simulink model "sat_CH_MC_v7"  (R2017b)
settings: Solver=VariableStepAuto  StartTime=0.0  StopTime=2000  RelTol=1e-5
settings Model: Creator=J  LastModifiedBy=student

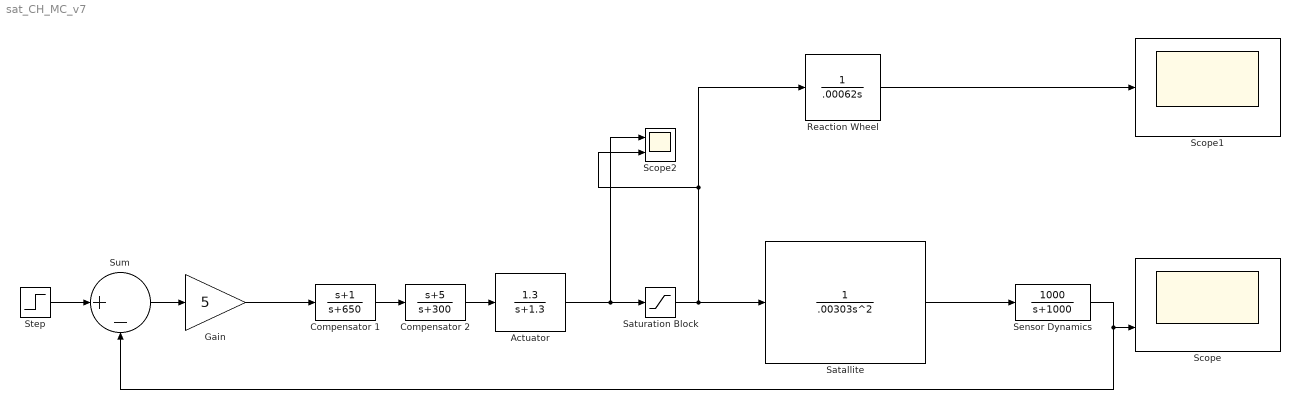
== system sat_CH_MC_v7 ==
  Actuator : TransferFcn  Numerator=[1.3]  Denominator=[1 1.3]
  Compensator 1 : TransferFcn  Numerator=[1 1]  Denominator=[1 650]
  Compensator 2 : TransferFcn  Numerator=[1 5]  Denominator=[1 300]
  Gain : Gain  Gain=5
  Reaction Wheel : TransferFcn  Denominator=[.00062 0]
  Satallite : TransferFcn  Denominator=[.00303 0 0]
  Saturation Block : Saturate  UpperLimit=.007  LowerLimit=-.007
  Scope : Scope  NumInputPorts=2
  Scope1 : Scope
  Scope2 : Scope  NumInputPorts=2
  Sensor Dynamics : TransferFcn  Numerator=[1000]  Denominator=[1 1000]
  Step : Step  SampleTime=0
  Sum : Sum  Inputs=|+-
  wires:
  Actuator/1 -> Scope2/1, Saturation Block/1
  Sum/1 -> Gain/1
  Step/1 -> Sum/1
  Saturation Block/1 -> Satallite/1, Reaction Wheel/1, Scope2/2
  Reaction Wheel/1 -> Scope1/1
  Satallite/1 -> Sensor Dynamics/1
  Sensor Dynamics/1 -> Sum/2, Scope/2
  Gain/1 -> Compensator 1/1
  Compensator 2/1 -> Actuator/1
  Compensator 1/1 -> Compensator 2/1
